simulink model "neurocircle"  (Simulink 8.3)
settings: Solver=ode3  StartTime=0.0  StopTime=1500  FixedStep=0.3  MinStep=0.1  RelTol=1e-3
libraries: simulink x1
settings Model: Creator=Administrator  LastModifiedBy=hasee
settings OptimizationCC: ExpressionDepthLimit=2147483647
settings DebuggingCC: FcnCallInpInsideContextMsg=UseLocalSettings

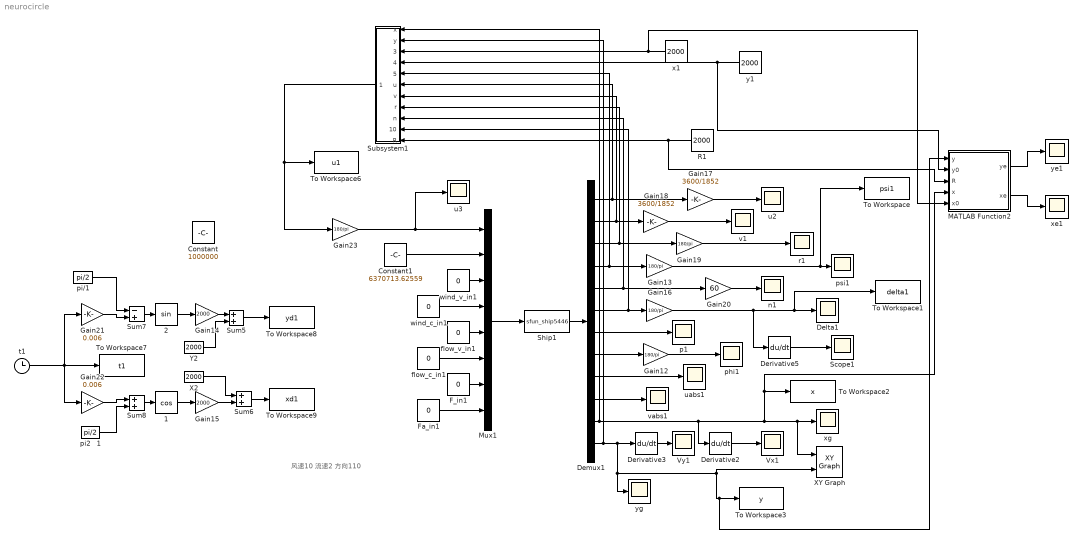
== system neurocircle ==
  note: 风速10 流速2 方向110
  "  2" : Trigonometry
  " 1" : Trigonometry  Operator=cos
  Constant : Constant  Value=1000000
  Constant1 : Constant  Value=6370713.62559
  Delta1 : Scope
      settings: TickLabels=on  TimeRange=1500  YMin=-20  YMax=12.5  SaveName=ScopeData5
  Demux1 : Demux  Outputs=12
  Derivative2 : Derivative
  Derivative3 : Derivative
  Derivative5 : Derivative
  F_in1 : Constant  Value=0
  Fa_in1 : Constant  Value=0
  Gain{12..13,16,19,23} (5 alike) : Gain  Gain=180/pi
  Gain14 : Gain  Gain=2000
  Gain15 : Gain  Gain=2000
  Gain17 : Gain  Gain=3600/1852
  Gain18 : Gain  Gain=3600/1852
  Gain20 : Gain  Gain=60
  Gain21 : Gain  Gain=0.006
  Gain22 : Gain  Gain=0.006
  MATLAB Function2 : MATLAB Function  TreatAsAtomicUnit=on
  Mux1 : Mux  Inputs=8
  R1 : Constant  Value=2000
  Scope1 : Scope
      settings: YMin=-0.005  YMax=0.002  SaveName=ScopeData31
  Ship1 : S-Function  FunctionName=sfun_ship5446  EnableBusSupport=off
  Subsystem1 : Subsystem
  Sum5 : Sum
  Sum6 : Sum
  Sum7 : Sum  Inputs=-+
  Sum8 : Sum
  To Workspace : ToWorkspace  VariableName=psi1  SampleTime=-1
  To Workspace1 : ToWorkspace  VariableName=delta1  SampleTime=-1
  To Workspace2 : ToWorkspace  VariableName=x  SampleTime=-1
  To Workspace3 : ToWorkspace  VariableName=y  SampleTime=-1
  To Workspace6 : ToWorkspace  VariableName=u1  SampleTime=-1
  To Workspace7 : ToWorkspace  VariableName=t1  SampleTime=-1
  To Workspace8 : ToWorkspace  VariableName=yd1  SampleTime=-1
  To Workspace9 : ToWorkspace  VariableName=xd1  SampleTime=-1
  Vx1 : Scope
      settings: TickLabels=on  SaveName=ScopeData32
  Vy1 : Scope
      settings: TickLabels=on  SaveName=ScopeData33
  X2 : Constant  Value=2000
  XY Graph : simulink/Sinks/XY Graph  xmin=-1000  xmax=5000  ymin=-1000  ymax=5000  st=-1
  Y2 : Constant  Value=2000
  flow_c_in1 : Constant  Value=0
  flow_v_in1 : Constant  Value=0
  n1 : Scope
      settings: TickLabels=on  YMin=38.5  YMax=46.5  SaveName=ScopeData34
  p1 : Scope
      settings: TickLabels=on  SaveName=ScopeData35
  phi1 : Scope
      settings: YMin=-0.00175  YMax=0.0015  SaveName=ScopeData36
  pi/1 : Constant  Value=pi/2
  pi2   1 : Constant  Value=pi/2
  psi1 : Scope
      settings: TickLabels=on  TimeRange=44.44444444444434  YMin=52  YMax=60.5  SaveName=ScopeData3
  r1 : Scope
      settings: TickLabels=on  SaveName=ScopeData37
  t1 : Clock
  u2 : Scope
      settings: TickLabels=on  YMin=28.45  YMax=29.45  SaveName=ScopeData38
  u3 : Scope
      settings: TickLabels=on  TimeRange=1500  YMin=-35000  YMax=35000  SaveName=ScopeData15
  uabs1 : Scope
      settings: TickLabels=on  YMin=10.75  YMax=15  SaveName=ScopeData39
  v1 : Scope
      settings: TickLabels=on  SaveName=ScopeData40
  vabs1 : Scope
      settings: TickLabels=on  YMin=-1.75  YMax=0  SaveName=ScopeData41
  wind_c_in1 : Constant  Value=0
  wind_v_in1 : Constant  Value=0
  x1 : Constant  Value=2000
  xe1 : Scope
      settings: TickLabels=on  YMin=-475  YMax=50  SaveName=ScopeData42
  xg : Scope
      settings: TickLabels=on  YMin=250  YMax=475  SaveName=ScopeData12
  y1 : Constant  Value=2000
  ye1 : Scope
      settings: TickLabels=on  YMin=-550  YMax=250  SaveName=ScopeData43
  yg : Scope
      settings: TickLabels=on  YMin=250  YMax=475  SaveName=ScopeData13
  wires:
  Ship1/1 -> Demux1/1
  Demux1/1 -> Subsystem1/6(u), Gain17/1
  Demux1/2 -> Subsystem1/7(v), Gain18/1
  Demux1/3 -> Subsystem1/8(r), Gain19/1
  Demux1/5 -> Subsystem1/9(n), Gain20/1
  Demux1/7 -> p1/1
  Demux1/8 -> Gain12/1
  Demux1/4 -> Gain13/1, Subsystem1/5(psi)
  Gain12/1 -> phi1/1
  Gain16/1 -> Derivative5/1, Delta1/1, To Workspace1/1
  Gain17/1 -> u2/1
  Gain18/1 -> v1/1
  Gain19/1 -> r1/1
  Gain20/1 -> n1/1
  Demux1/9 -> uabs1/1
  Demux1/10 -> vabs1/1
  Demux1/12 -> Subsystem1/2(y), Derivative3/1, yg/1, MATLAB Function2/1(y), To Workspace3/1, XY Graph/2
  Demux1/11 -> Subsystem1/1(x), Derivative2/1, XY Graph/1, xg/1, MATLAB Function2/4(x), To Workspace2/1
  Derivative2/1 -> Vx1/1
  Derivative3/1 -> Vy1/1
  wind_v_in1/1 -> Mux1/3
  wind_c_in1/1 -> Mux1/4
  flow_v_in1/1 -> Mux1/5
  F_in1/1 -> Mux1/7
  Fa_in1/1 -> Mux1/8
  flow_c_in1/1 -> Mux1/6
  Mux1/1 -> Ship1/1
  Constant1/1 -> Mux1/2
  Derivative5/1 -> Scope1/1
  Gain23/1 -> u3/1, Mux1/1
  y1/1 -> MATLAB Function2/2(y0), Subsystem1/4(y0)
  R1/1 -> MATLAB Function2/3(R), Subsystem1/11(R)
  Sum5/1 -> To Workspace8/1
  "  2"/1 -> Gain14/1
  " 1"/1 -> Gain15/1
  t1/1 -> To Workspace7/1, Gain22/1, Gain21/1
  Gain14/1 -> Sum5/1
  Gain15/1 -> Sum6/2
  X2/1 -> Sum6/1
  Y2/1 -> Sum5/2
  Sum7/1 -> "  2"/1
  Gain21/1 -> Sum7/2
  pi/1/1 -> Sum7/1
  Sum8/1 -> " 1"/1
  Gain22/1 -> Sum8/1
  pi2   1/1 -> Sum8/2
  Demux1/6 -> Subsystem1/10(Delta), Gain16/1
  Subsystem1/1("psi ") -> To Workspace6/1, Gain23/1
  MATLAB Function2/2(xe) -> xe1/1
  MATLAB Function2/1(ye) -> ye1/1
  x1/1 -> MATLAB Function2/5(x0), Subsystem1/3(x0)
  Gain13/1 -> psi1/1, To Workspace/1
  Sum6/1 -> To Workspace9/1

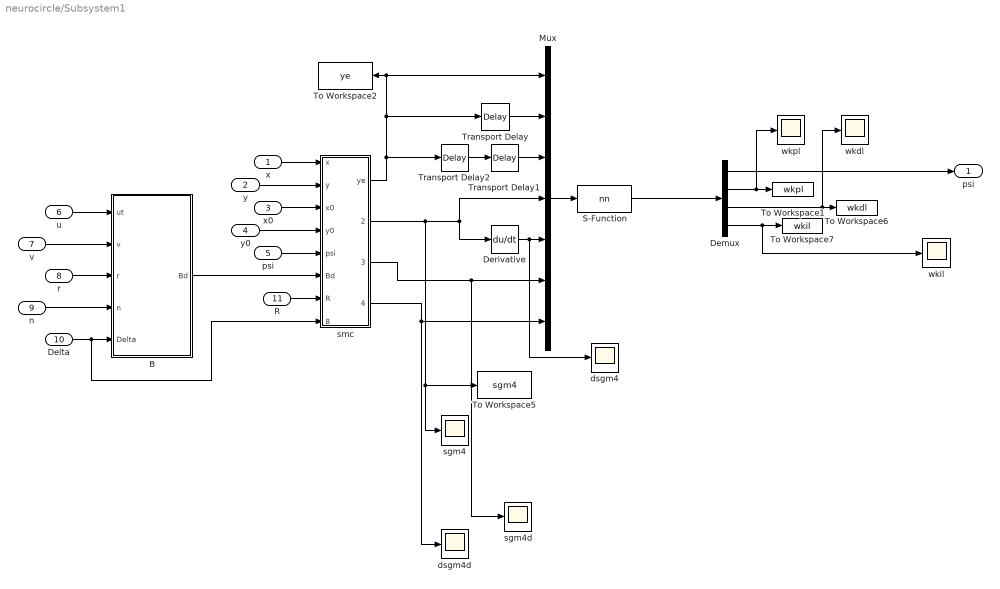
== system neurocircle/Subsystem1 ==
  x : Inport
  y : Inport  Port=2
  x0 : Inport  Port=3
  y0 : Inport  Port=4
  psi : Inport  Port=5
  u : Inport  Port=6
  v : Inport  Port=7
  r : Inport  Port=8
  n : Inport  Port=9
  Delta : Inport  Port=10
  R : Inport  Port=11
  B : MATLAB Function  TreatAsAtomicUnit=on
  Demux : Demux
  Derivative : Derivative
  Mux : Mux  Inputs=7
  S-Function : S-Function  FunctionName=nn  EnableBusSupport=off
  To Workspace1 : ToWorkspace  VariableName=wkpl  SampleTime=-1
  To Workspace2 : ToWorkspace  VariableName=ye  SampleTime=-1
  To Workspace5 : ToWorkspace  VariableName=sgm4  SampleTime=-1
  To Workspace6 : ToWorkspace  VariableName=wkdl  SampleTime=-1
  To Workspace7 : ToWorkspace  VariableName=wkil  SampleTime=-1
  Transport Delay : TransportDelay  DelayTime=2
  Transport Delay1 : TransportDelay
  Transport Delay2 : TransportDelay
  dsgm4 : Scope
      settings: TickLabels=on  TimeRange=1500  YMin=-4.20046e+11  YMax=-3.80042e+11  SaveName=ScopeData25
  dsgm4d : Scope
      settings: TickLabels=on  TimeRange=1500  YMin=0.00019  YMax=0.00028  SaveName=ScopeData23
  sgm4 : Scope
      settings: TickLabels=on  TimeRange=1500  YMin=-0.0004  YMax=0.0004  SaveName=ScopeData24
  sgm4d : Scope
      settings: TickLabels=on  TimeRange=1500  YMin=0.00975  YMax=0.014  SaveName=ScopeData21
  "smc " : Subsystem
  wkdl : Scope
      settings: TickLabels=on  TimeRange=1500  YMin=0.3  YMax=1  SaveName=ScopeData19
  wkil : Scope
      settings: TickLabels=on  TimeRange=1500  YMin=-0.025  YMax=0.35  SaveName=ScopeData20
  wkpl : Scope
      settings: TickLabels=on  TimeRange=1500  YMin=-0.3  YMax=0.5  SaveName=ScopeData22
  "psi " : Outport
  wires:
  x/1 -> "smc "/1(x)
  y/1 -> "smc "/2(y)
  x0/1 -> "smc "/3(x0)
  y0/1 -> "smc "/4(y0)
  psi/1 -> "smc "/5("psi ")
  u/1 -> B/1(ut)
  v/1 -> B/2(v)
  r/1 -> B/3(r)
  n/1 -> B/4(n)
  Mux/1 -> S-Function/1
  Transport Delay/1 -> Mux/2
  Transport Delay1/1 -> Mux/3
  Derivative/1 -> dsgm4/1, Mux/5
  B/1(Bd) -> "smc "/6(Bd)
  Transport Delay2/1 -> Transport Delay1/1
  R/1 -> "smc "/7(R)
  Delta/1 -> "smc "/8(delta), B/5(Delta)
  S-Function/1 -> Demux/1
  Demux/2 -> To Workspace1/1, wkpl/1
  Demux/3 -> To Workspace6/1, wkdl/1
  Demux/4 -> wkil/1, To Workspace7/1
  Demux/1 -> "psi "/1
  "smc "/1(ye) -> Transport Delay2/1, Transport Delay/1, Mux/1, To Workspace2/1
  "smc "/2(sgm4) -> Mux/4, Derivative/1, To Workspace5/1, sgm4/1
  "smc "/3(sgm4d) -> sgm4d/1, Mux/6
  "smc "/4(dsgm4d) -> Mux/7, dsgm4d/1

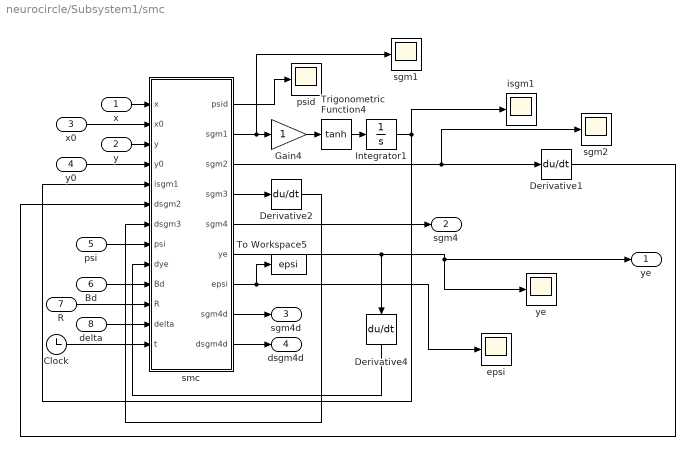
== system neurocircle/Subsystem1/smc  ==
  x : Inport
  y : Inport  Port=2
  x0 : Inport  Port=3
  y0 : Inport  Port=4
  "psi " : Inport  Port=5
  Bd : Inport  Port=6
  R : Inport  Port=7
  delta : Inport  Port=8
  Clock : Clock
  Derivative1 : Derivative
  Derivative2 : Derivative
  Derivative4 : Derivative
  Gain4 : Gain
  Integrator1 : Integrator
  To Workspace5 : ToWorkspace  VariableName=epsi  SampleTime=-1
  Trigonometric Function4 : Trigonometry  Operator=tanh
  epsi : Scope
      settings: TickLabels=on  TimeRange=1500  YMin=-0.1  YMax=0.8  SaveName=ScopeData29
  isgm1 : Scope
      settings: TickLabels=on  TimeRange=1500  YMin=-150  YMax=650  SaveName=ScopeData28
  psid : Scope
      settings: TickLabels=on  TimeRange=1500  YMin=-3.5  YMax=3.5  SaveName=ScopeData30
  sgm1 : Scope
      settings: TickLabels=on  TimeRange=1500  YMin=-15  YMax=15  SaveName=ScopeData26
  sgm2 : Scope
      settings: TickLabels=on  TimeRange=1500  YMax=7  SaveName=ScopeData27
  "smc " : MATLAB Function  TreatAsAtomicUnit=on
  "ye " : Scope
      settings: TimeRange=1500  YMin=-300  YMax=850  SaveName=ScopeData14
  ye : Outport
  sgm4 : Outport  Port=2
  sgm4d : Outport  Port=3
  dsgm4d : Outport  Port=4
  wires:
  "smc "/2(sgm1) -> sgm1/1, Gain4/1
  Derivative2/1 -> "smc "/7(dsgm3)
  "smc "/4(sgm3) -> Derivative2/1
  Trigonometric Function4/1 -> Integrator1/1
  Derivative1/1 -> "smc "/6(dsgm2)
  Integrator1/1 -> isgm1/1, "smc "/5(isgm1)
  x/1 -> "smc "/1(x)
  y/1 -> "smc "/3(y)
  x0/1 -> "smc "/2(x0)
  y0/1 -> "smc "/4(y0)
  "smc "/5(sgm4) -> sgm4/1
  "smc "/6(ye) -> "ye "/1, ye/1, Derivative4/1
  Bd/1 -> "smc "/10(Bd)
  Derivative4/1 -> "smc "/9(dye)
  "smc "/8(sgm4d) -> sgm4d/1
  "smc "/9(dsgm4d) -> dsgm4d/1
  R/1 -> "smc "/11(R)
  delta/1 -> "smc "/12(delta)
  "smc "/7(epsi) -> To Workspace5/1, epsi/1
  Gain4/1 -> Trigonometric Function4/1
  "smc "/1(psid) -> psid/1
  "psi "/1 -> "smc "/8(psi)
  "smc "/3(sgm2) -> Derivative1/1, sgm2/1
  Clock/1 -> "smc "/13(t)

== matlab function MATLAB Function2 ==
  data: y input double; ye output double; y0 input double; R input double; x input double; x0 input double; xe output double
function [ye,xe]= fcn(y,y0,R,x,x0)
%#codegen

thta=atan2((y-y0),(x-x0));
xe = x-x0-R*cos(thta);
ye = y-y0-R*sin(thta);

== matlab function Subsystem1/B ==
  data: ut input double; Bd output double; v input double; r input double; n input double; Delta input double
%%%%%%%%%%%%%%%%%%%%%%%%%%%%%%%%%%%%%%%%%%%%%%%%%%%%%%%%%%%%%
%%源自: 沈智鹏 著《船舶运动自适应滑模控制》 2019年科学出版社
%%下载地址www.shenbert.cn/book/shipmotionASMC.html
%%%%%%%%%%%%%%%%%%%%%%%%%%%%%%%%%%%%%%%%%%%%%%%%%%%%%%%%%%%%%%
function Bd  = fcn(ut,v,r,n,Delta)
% function ud = fcn(ut,v,r,n,Delta,phi,dr,sgm4)
V=sqrt(ut*ut+v*v);%u=x(1) v=x(2)

da=10.5;%9.34+0.25;%尾吃水13.8;%12.5;%
df=7.5;%4.97+0.25;%首吃水14.3;%13.8;%
Dh=9.0;%舵高s   ;%11.411.4;;%+7.00+0.25
pa=1.205;%%%**空气密度
Lpp=267.0;%船长
B=39.8;%船宽
Db=6.466;%舵宽
P=9.657;%da螺距
luow=1026;%小luow是密度 水密度
Dp=9.2;%螺旋桨直径
Ds=23.6;%型深
d=(da+df)/2;%吃水
m=(165.89*d*d + 4383.9*d)*1000;%排水量
Cb=m/(Lpp*B*d*1.025*1000);
AR=(d-7.41)/(12.5-7.41)*(81.44-43.14)+43.14;%舵叶面积
d_B=d/B;L_B=Lpp/B;
mx=m/100*(0.398+11.97*Cb*(1+3.73*d_B)-2.89*Cb*L_B*(1+1.13*d_B)+0.175*Cb*L_B*L_B*(1+0.541*d_B)-1.107*L_B*d_B);
my=m*(0.882-0.54*Cb*(1-1.6*d_B)-0.156*L_B*(1-0.673*Cb)+0.826*d_B*L_B*(1-0.678*d_B)-0.638*Cb*d_B*L_B*(1-0.669*d_B));
wp0=0.5*Cb-0.05;
fa=6.13*Dh/Db/(2.25+Dh/Db);
gma=-22.2*(Cb*B/Lpp)*(Cb*B/Lpp)+0.02*(Cb*B/Lpp)+0.68;
gmaR=1.1633-1.98828*Cb+1.3902*Cb*Cb;
tR=0.7382-0.0539*Cb+0.1755*Cb*Cb;
ifaH=0.6784-1.3374*Cb+1.8891*Cb*Cb;
xH=-(0.4+0.1*Cb)*Lpp;
xR=-0.5*Lpp;
xb=1.87;
Jzz=1/100.0*(33-76.85*Cb*(1-0.784*Cb)+3.43*L_B*(1-0.63*Cb))*Lpp*Lpp;
Izz=(1.0+(Cb^4.5))*m*(Lpp*Lpp+power(B,2.4))/24.0;

m33=Izz+Jzz;

beta=atan2((-v),(ut));%u=x(1) v=x(2)
betap=beta+0.5*r*Lpp/V;%r=x(3)
betaR=beta+r*Lpp/V;
wp=wp0*exp(-4.0*betap*betap);
up=(1.0-wp)*ut;%u=x(1)
s=1.0-up/n/P;% n=x(5)
eta=Dp/Dh;

k=0.6;
Gs=eta*k*(2.0-(2.0-k)*s)*s/(1.0-s)/(1.0-s);
s0=1-(1-wp0)*ut/n/P;% n=x(5)u=x(1)
delt0=-s0/57.3;

if(Delta<0)
    K=1.065;
else
    K=0.935;
end
%
uR=up*(1+K*Gs)^0.5;
vRp=uR*delt0;
vR=vRp-gmaR*(v-Lpp*r);%r=x(3)v=x(2)
UR2=uR*uR+vR*vR;
J=ut*(1-wp)/n/Dp;%u=x(1)  n=x(5)
if(J<=0.3)
    L_ifaH=ifaH*J/0.3;% p137, 3-5-119
else
    L_ifaH=ifaH;
end
%
Bd=(-1.0/2.0)*(xR+L_ifaH*xH)*luow*AR*fa*UR2*cos(Delta)/(m33);

== matlab function Subsystem1/smc /smc  ==
  data: psid output double; x input double; x0 input double; y input double; y0 input double; isgm1 input double; dsgm2 input double; dsgm3 input double; sgm1 output double; sgm2 output double; sgm3 output double; psi input double; dye input double; sgm4 output double; ye output double; epsi output double; Bd input double; sgm4d output double; dsgm4d output double; R input double; delta input double; t input double
function [psid,sgm1,sgm2,sgm3,sgm4,ye,epsi,sgm4d,dsgm4d]= fcn(x,x0,y,y0,isgm1,dsgm2,dsgm3,psi,dye,Bd,R,delta,t)
%#codegen
k0=1;k1=4;k2=0.0000001;k3=0.0000001;k4=0.03;
%k0=0.8;k1=0.001;k2=0.0000001;k3=0.0000002;k4=0.04;
 ye=sqrt((x-x0)^2+(y-y0)^2)-R;
if(atan2((y-y0),(x-x0))<0&&t>700)
    epsi=psi-atan2((y-y0),(x-x0))-pi/2-2*pi;
elseif(atan2((y-y0),(x-x0))>0&&t>1000)
    epsi=psi-atan2((y-y0),(x-x0))-pi/2-2*pi;
else
    epsi=psi-atan2((y-y0),(x-x0))-pi/2;     
end

  psid=atan2((y-y0),(x-x0));
% if(t<=784.2)
%   epsi=psi-psid-pi/2;
% else
%   epsi=0.0473;
% end
% epsi=psi-psid-pi/2;
sgm1=k1*tanh(k0*ye)+dye;
sgm2=epsi+k2*isgm1;
sgm3=k3*tanh(sgm2)+dsgm2;
sgm4=k4*tanh(sgm3)+dsgm3;

sgm4d=Bd; 
dsgm4d=(k4*(sech(sgm3)^2)+k3*(sech(sgm2)^2))*Bd;
